simulink model "PosControl_Quadruped_v3_attitude"  (R2018b)
settings: Solver=FixedStepAuto  StartTime=0.0  StopTime=10  FixedStep=0.001  RelTol=1e-3  EnableMultiTasking=on
undefined symbols (not defined in the file or in its folder): X, Y, Z
libraries: sm_lib x43, nesl_utility x39, Contact_Forces_Lib x4
(part 3 of 3)

== matlab function PosControl_Quadruped_v3_attitude/controller/trajectory generate1 ==
  data: timer1 input; timer2 input; timer1 output; timer2 output; roll input; pitch input; yaw input; LegFL output; LegFR output; LegRR output; LegRL output
function [timer1,timer2,LegFL,LegFR,LegRR,LegRL] = gesture( timer1,timer2,roll,pitch,yaw)

if timer2<2
    timer2 = timer2+0.001;
else
    timer1 = timer1+0.002;
end

Xs = 0;
Ys = 0;
Zs = -0.7;

if timer1>0
    O_FL = [0.6,0.25,-0.7,1]';
    O_FR = [0.6,-0.25,-0.7,1]';
    O_RR = [-0.6,-0.25,-0.7,1]';
    O_RL = [-0.6,0.25,-0.7,1]';
    
    FL = [0.6,0.25,0]';
    FR = [0.6,-0.25,0]';
    RR = [-0.6,-0.25,0]';
    RL = [-0.6,0.25,0]';
    
    FL_trans = [eye(3,3),FL;
        zeros(1,3),1];
    FR_trans = [eye(3,3),FR;
        zeros(1,3),1];
    RR_trans = [eye(3,3),RR;
        zeros(1,3),1];
    RL_trans = [eye(3,3),RL;
        zeros(1,3),1];
    
    R_roll = [ 1,0,0,0;
        0,cos(roll),-sin(roll),0;
        0,sin(roll),cos(roll),0;
        0,0,0,1];
    
    R_pitch = [cos(pitch),0,sin(pitch),0;
        0,1,0,0;
        -sin(pitch),0,cos(pitch),0;
        0,0,0,1];
    
    R_yaw = [cos(yaw),-sin(yaw),0,0;
        sin(yaw),cos(yaw),0,0;
        0,0,1,0;
        0,0,0,1];
    
    
%     P_FL_roll = inv(FL_trans)*R_roll*O_FL;
%     P_FL_pitch = inv(FL_trans)*R_pitch*O_FL;
%     P_FL_yaw = inv(FL_trans)*R_yaw*O_FL;
%     
%     P_FR_roll = inv(FR_trans)*R_roll*O_FR;
%     P_FR_pitch = inv(FR_trans)*R_pitch*O_FR;
%     P_FR_yaw = inv(FR_trans)*R_yaw*O_FR;
%     
%     P_RR_roll = inv(RR_trans)*R_roll*O_RR;
%     P_RR_pitch = inv(RR_trans)*R_pitch*O_RR;
%     P_RR_yaw = inv(RR_trans)*R_yaw*O_RR;
%     
%     P_RL_roll = inv(RL_trans)*R_roll*O_RL;
%     P_RL_pitch = inv(RL_trans)*R_pitch*O_RL;
%     P_RL_yaw = inv(RL_trans)*R_yaw*O_RL;
    
    P_FL_all = inv(FL_trans)*R_roll*R_pitch*R_yaw*O_FL;
    P_FR_all = inv(FR_trans)*R_roll*R_pitch*R_yaw*O_FR;
    P_RR_all = inv(RR_trans)*R_roll*R_pitch*R_yaw*O_RR;
    P_RL_all = inv(RL_trans)*R_roll*R_pitch*R_yaw*O_RL;
    
    
%     LegFL = P_FL_roll(1:3)';
%     LegFR = P_FR_roll(1:3)';
%     LegRR = P_RR_roll(1:3)';
%     LegRL = P_RL_roll(1:3)';
    
%     LegFL = P_FL_pitch(1:3)';
%     LegFR = P_FR_pitch(1:3)';
%     LegRR = P_RR_pitch(1:3)';
%     LegRL = P_RL_pitch(1:3)';

%     LegFL = P_FL_yaw(1:3)';
%     LegFR = P_FR_yaw(1:3)';
%     LegRR = P_RR_yaw(1:3)';
%     LegRL = P_RL_yaw(1:3)';

    LegFL = P_FL_all(1:3)';
    LegFR = P_FR_all(1:3)';
    LegRR = P_RR_all(1:3)';
    LegRL = P_RL_all(1:3)';
else
    LegFL = [Xs,Ys,Zs];
    LegFR = [Xs,Ys,Zs];
    LegRR = [Xs,Ys,Zs];
    LegRL = [Xs,Ys,Zs];
end

== matlab function PosControl_Quadruped_v3_attitude/controller/inverse kinematics2 ==
  data: x input; y input; z input; shoulder output; hip output; knee output
function [shoulder,hip,knee]= coord2theta(x,y,z)
% L1=75.0;
% L2=415.0;
% L3=408.0;


% temp = (L1*L1+L2*L2-x*x-z*z)/(2*L1*L2);
% if temp>1
%     temp = 1;
% elseif temp<-1
%     temp=1;
% end
% theta2 = pi-acos(temp);
% 
% temp = (x*x+z*z+L1*L1-L2*L2)/(2*sqrt(x*x+z*z)*L1);
% if temp>1
%     temp = 1;
% elseif temp<-1
%     temp=1;
% end
% if(x>0)
%     theta1 = abs(atan(x/z))-acos(temp);
% elseif(x<0)
%     theta1 = -abs(atan(x/z))-acos(temp);
% else
%     theta1 = -acos(temp);

L1=0;
L2=0.5;
L3=0.5;

shoulder=atan(-y/z);

%髋关节到足端长度的平方
L_H2E_2=x*x+(y-L1*sin(shoulder))*(y-L1*sin(shoulder))+(z+L1*cos(shoulder))*(z+L1*cos(shoulder));
%髋关节到足端长度
L_H2E=sqrt(L_H2E_2);

temp = (L2*L2+L_H2E_2-L3*L3)/(2*L_H2E*L2);
if temp>1
    temp = 1;
elseif temp<-1
    temp = -1;
end
Zeta=acos(temp);
hip=atan(x/(sqrt(y*y+z*z)-L1))-Zeta;

temp = (L2*L2+L3*L3-L_H2E_2)/(2*L2*L3);
if temp>1
    temp = 1;
elseif temp<-1
    temp = -1;
end
knee=pi-acos(temp);

== matlab function PosControl_Quadruped_v3_attitude/controller/inverse kinematics3 ==
  data: x input; y input; z input; shoulder output; hip output; knee output
function [shoulder,hip,knee]= coord2theta(x,y,z)
% L1=75.0;
% L2=415.0;
% L3=408.0;


% temp = (L1*L1+L2*L2-x*x-z*z)/(2*L1*L2);
% if temp>1
%     temp = 1;
% elseif temp<-1
%     temp=1;
% end
% theta2 = pi-acos(temp);
% 
% temp = (x*x+z*z+L1*L1-L2*L2)/(2*sqrt(x*x+z*z)*L1);
% if temp>1
%     temp = 1;
% elseif temp<-1
%     temp=1;
% end
% if(x>0)
%     theta1 = abs(atan(x/z))-acos(temp);
% elseif(x<0)
%     theta1 = -abs(atan(x/z))-acos(temp);
% else
%     theta1 = -acos(temp);

L1=0;
L2=0.5;
L3=0.5;

shoulder=atan(-y/z);

%髋关节到足端长度的平方
L_H2E_2=x*x+(y-L1*sin(shoulder))*(y-L1*sin(shoulder))+(z+L1*cos(shoulder))*(z+L1*cos(shoulder));
%髋关节到足端长度
L_H2E=sqrt(L_H2E_2);

temp = (L2*L2+L_H2E_2-L3*L3)/(2*L_H2E*L2);
if temp>1
    temp = 1;
elseif temp<-1
    temp = -1;
end
Zeta=acos(temp);
hip=atan(x/(sqrt(y*y+z*z)-L1))-Zeta;

temp = (L2*L2+L3*L3-L_H2E_2)/(2*L2*L3);
if temp>1
    temp = 1;
elseif temp<-1
    temp = -1;
end
knee=pi-acos(temp);

== matlab function PosControl_Quadruped_v3_attitude/controller/inverse kinematics4 ==
  data: x input; y input; z input; shoulder output; hip output; knee output
function [shoulder,hip,knee]= coord2theta(x,y,z)
% L1=75.0;
% L2=415.0;
% L3=408.0;


% temp = (L1*L1+L2*L2-x*x-z*z)/(2*L1*L2);
% if temp>1
%     temp = 1;
% elseif temp<-1
%     temp=1;
% end
% theta2 = pi-acos(temp);
% 
% temp = (x*x+z*z+L1*L1-L2*L2)/(2*sqrt(x*x+z*z)*L1);
% if temp>1
%     temp = 1;
% elseif temp<-1
%     temp=1;
% end
% if(x>0)
%     theta1 = abs(atan(x/z))-acos(temp);
% elseif(x<0)
%     theta1 = -abs(atan(x/z))-acos(temp);
% else
%     theta1 = -acos(temp);

L1=0;
L2=0.5;
L3=0.5;

shoulder=atan(-y/z);

%髋关节到足端长度的平方
L_H2E_2=x*x+(y-L1*sin(shoulder))*(y-L1*sin(shoulder))+(z+L1*cos(shoulder))*(z+L1*cos(shoulder));
%髋关节到足端长度
L_H2E=sqrt(L_H2E_2);

temp = (L2*L2+L_H2E_2-L3*L3)/(2*L_H2E*L2);
if temp>1
    temp = 1;
elseif temp<-1
    temp = -1;
end
Zeta=acos(temp);
hip=atan(x/(sqrt(y*y+z*z)-L1))-Zeta;

temp = (L2*L2+L3*L3-L_H2E_2)/(2*L2*L3);
if temp>1
    temp = 1;
elseif temp<-1
    temp = -1;
end
knee=pi-acos(temp);

== matlab function PosControl_Quadruped_v3_attitude/controller/inverse kinematics5 ==
  data: x input; y input; z input; shoulder output; hip output; knee output
function [shoulder,hip,knee]= coord2theta(x,y,z)
% L1=75.0;
% L2=415.0;
% L3=408.0;


% temp = (L1*L1+L2*L2-x*x-z*z)/(2*L1*L2);
% if temp>1
%     temp = 1;
% elseif temp<-1
%     temp=1;
% end
% theta2 = pi-acos(temp);
% 
% temp = (x*x+z*z+L1*L1-L2*L2)/(2*sqrt(x*x+z*z)*L1);
% if temp>1
%     temp = 1;
% elseif temp<-1
%     temp=1;
% end
% if(x>0)
%     theta1 = abs(atan(x/z))-acos(temp);
% elseif(x<0)
%     theta1 = -abs(atan(x/z))-acos(temp);
% else
%     theta1 = -acos(temp);

L1=0;
L2=0.5;
L3=0.5;

shoulder=atan(-y/z);

%髋关节到足端长度的平方
L_H2E_2=x*x+(y-L1*sin(shoulder))*(y-L1*sin(shoulder))+(z+L1*cos(shoulder))*(z+L1*cos(shoulder));
%髋关节到足端长度
L_H2E=sqrt(L_H2E_2);

temp = (L2*L2+L_H2E_2-L3*L3)/(2*L_H2E*L2);
if temp>1
    temp = 1;
elseif temp<-1
    temp = -1;
end
Zeta=acos(temp);
hip=atan(x/(sqrt(y*y+z*z)-L1))-Zeta;

temp = (L2*L2+L3*L3-L_H2E_2)/(2*L2*L3);
if temp>1
    temp = 1;
elseif temp<-1
    temp = -1;
end
knee=pi-acos(temp);

== matlab function PosControl_Quadruped_v3_attitude/controller/trajectory generate2 ==
  data: t input; xLegFL output; yLegFL output; zLegFL output; xLegFR output; yLegFR output; zLegFR output; xLegRR output; yLegRR output; zLegRR output; xLegRL output; yLegRL output; zLegRL output
function [xLegFL,yLegFL,zLegFL,xLegFR,yLegFR,zLegFR,xLegRR,yLegRR,zLegRR,xLegRL,yLegRL,zLegRL] = Turn(t)

lamda = 0.5;%摆动周期占比
Ts = 1;%周期时间

Xs = -0.1;%x轴起点
Xe = -0.1;%x轴终点

Ys = 0;%y轴起点
YeR = -0.05;%y轴右转终点

H = 0.2;%抬腿高度
Zs = -0.7;%z轴起点

if t>0 && t<=lamda*Ts
    sigma = 2*pi*t/(lamda*Ts);
    
    x2f = (Xe-Xs)*((sigma-sin(sigma))/(2*pi))+Xs;
    x2b = (Xs-Xe)*((sigma-sin(sigma))/(2*pi))+Xe;
    
%     y_O2R =  (YeR-Ys)*((sigma-sin(sigma))/(2*pi))+Ys;
%     y_O2L =  -y_O2R;
%     
%     y_R2O = (Ys-YeR)*((sigma-sin(sigma))/(2*pi))+YeR;
%     y_L2O = -y_R2O;
       
    zUP = H*(1-cos(sigma))/2+Zs;
   
    xLegFL = x2f;
    yLegFL = Ys;
    zLegFL = zUP;
    
    xLegFR = x2b;
    yLegFR = Ys;
    zLegFR = Zs;
    
    xLegRR = x2f;
    yLegRR = Ys;
    zLegRR = zUP;
    
    xLegRL = x2b;
    yLegRL = Ys;
    zLegRL = Zs;
    
elseif t>lamda*Ts && t<Ts
    sigma = 2*pi*(t-lamda*Ts)/(lamda*Ts);
    
    x2f = (Xe-Xs)*((sigma-sin(sigma))/(2*pi))+Xs;
    x2b = (Xs-Xe)*((sigma-sin(sigma))/(2*pi))+Xe;
    
%     y_O2R =  (YeR-Ys)*((sigma-sin(sigma))/(2*pi))+Ys;
%     y_O2L =  -y_O2R;
%     
%     y_R2O = (Ys-YeR)*((sigma-sin(sigma))/(2*pi))+YeR;
%     y_L2O = -y_R2O;
    
    zUP = H*(1-cos(sigma))/2+Zs;
    
    xLegFL = x2b;
    yLegFL = Ys;
    zLegFL = Zs;
    
    xLegFR = x2f;
    yLegFR = Ys;
    zLegFR = zUP;
    
    xLegRR = x2b;
    yLegRR = Ys;
    zLegRR = Zs;
    
    xLegRL = x2f;
    yLegRL = Ys;
    zLegRL = zUP;
    
else
    xLegFL = Xs;
    yLegFL = Ys;
    zLegFL = Zs;
    
    xLegFR = Xs;
    yLegFR = Ys;
    zLegFR = Zs;
    
    xLegRR = Xs;
    yLegRR = Ys;
    zLegRR = Zs;
    
    xLegRL = Xs;
    yLegRL = Ys;
    zLegRL = Zs;
end
